simulink model "PropulsionTest"  (R2017b)
settings: Solver=FixedStepAuto  StartTime=0.0  StopTime=100*24*60*60  FixedStep=.2  RelTol=1e-3
model workspace: external: MATLAB File C:\Users\Justin\Documents\00 MEng Project\PAN_ADCS\initialization\simulink_workspace_init.m (data not in the file)
undefined symbols (not defined in the file): Imp_max, Imp_min, init, K_F, L_F, m_follower, match_tol, muE, ontime_max, ontime_min, Thrust_max, Thrust_min
libraries: hEemethod x8, vrlib x2, dspsigattribs x1
(part 2 of 2)

== matlab function PropulsionTest/Position and Velocity to Desired Attitude in Quat/dcm2quat ==
  data: DCM_be input; q output; tr output; q_prev input; flag output
function [q, tr, flag] = fcn(DCM_be,q_prev)
tr= DCM_be(1,1) + DCM_be(2,2) + DCM_be(3,3);
flag=[0 1];
if (tr > 0)
    S= sqrt(1+tr)*2;
    q4= 0.25 * S;
    q1= (DCM_be(3,2)-DCM_be(2,3))/S;
    q2= (DCM_be(1,3)-DCM_be(3,1))/S;
    q3= (DCM_be(2,1)-DCM_be(1,2))/S;
    q=[q1;q2;q3;q4];
    flag(1)=1;
    
elseif ((DCM_be(1,1)>DCM_be(2,2)) && (DCM_be(1,1)>DCM_be(3,3)))
    S= sqrt(1+DCM_be(1,1)-DCM_be(2,2)-DCM_be(3,3))*2;
    q4= (DCM_be(3,2)-DCM_be(2,3))/S;
    q1= 0.25*S;
    q2= (DCM_be(1,2)+DCM_be(2,1))/S;
    q3= (DCM_be(1,3)+DCM_be(3,1))/S;
    flag(1)=2;
    q=[q1;q2;q3;q4];
elseif (DCM_be(2,2)>DCM_be(3,3))
    S= sqrt(1+DCM_be(2,2)-DCM_be(1,1)-DCM_be(3,3))*2;
    q4= (DCM_be(1,3)-DCM_be(3,1))/S;
    q1= (DCM_be(1,2)+DCM_be(2,1))/S;
    q2= 0.25*S;
    q3= (DCM_be(2,3)+DCM_be(3,2))/S;
    flag(1)=3;
    q=[q1;q2;q3;q4];
else
    S= sqrt(1+DCM_be(3,3)-DCM_be(1,1)-DCM_be(2,2))*2;
    q4= (DCM_be(2,1)-DCM_be(1,2))/S;
    q1= (DCM_be(1,3)+DCM_be(3,1))/S;
    q2= (DCM_be(2,3)+DCM_be(3,2))/S;
    q3= 0.25*S;
    flag(1)=4;
    q=[q1;q2;q3;q4];
end


if  (flag(2)*sign(q(1))*sign(q_prev(1))==-1 && q(1)*q(1)>1e-8) || ...
    (flag(2)*sign(q(2))*sign(q_prev(2))==-1 && q(2)*q(2)>1e-8) || ...
    (flag(2)*sign(q(3))*sign(q_prev(3))==-1 && q(3)*q(3)>1e-8)
    %sign(q_prev(1))==0 || ...
    %sign(q_prev(2))==0 || ...
    %sign(q_prev(3))==0
    
    flag(2)=flag(2)*-1;
end
if flag(2)==-1
    q=-q;
end

== matlab function PropulsionTest/Subsystem/Propulsion/MATLAB Function ==
  data: Thrust_vectors output; Target input; onVec output
%%%Thrust Vector Calculations

%  Input: Vectorized Impulse Requirement (Target) [N*s], The Thrust Per Nozzle [N], and the thrust vectors on
%  the current nozzle block (Thrust_vectors, thought this is taken from
%  another function)

%  Output: Thruster On-time vector for the 3 main thrusters, the numbers of
%  the three main thrusters, the on time in terms of thrusters 1,2,3,4

% UNITS of this code is impulse, we take the force vectors of the nozzles
% then scale them accordingly
function [Thrust_vectors, onVec] = get_thruster_onTimes(Target)
%function [t_vector1stage, Best_3_names, onVec] = get_thruster_onTimes(Target,Thrust_per_nozzle)
    % check the input arguments
    [r,c] = size(Target);
    if r~=3 || c~=1
        error('Function argument must be a 3x1 vector')
    end
    % generate the thrust vectors based on the specific nozzle block and
    % the thrust measured per nozzle 
    
    %%% IMPUT THRUST PER NOZZLE %%%
    Thrust_vectors= zeros(3,4);
    Thrust_per_nozzle = 16E-3; %N
    [Thrust_vectors,~] = Generate_Thrust_Vectors(Thrust_per_nozzle); % generates 4x3 matrix 
    
        % determines thrust vectors to be used as a basis in the
        % firing
        angles = zeros(1,4);
        
        % check the angles to each thruster vector
        for i = 1:4 
            angles(i) = acos(dot(Thrust_vectors(:,i),Target)/(norm(Thrust_vectors(:,i))*norm(Target)));
            
        end

        [~,Indices] = sort(angles);
        Best_3_vectors = Thrust_vectors(:,Indices(1:3)); % loads the thruster's vectors
%         Best_2_vectors = Thrust_vectors(:,Indices(1:2));
%         Best_vector = Thrust_vectors(:,Indices(1));
        
        Best_3_names = [0 0 0];
        Best_3_names(1:3) = Indices(1:3); % loads names of the thrusters

        
   % generate on times (2 different methods)
   
   % method 1: 1 stage - 3 thrusters fire in one go, but for different
   % times each, the time vector t_vector1stage gives the thrust for the
   % associated thruster
        
        % x = A\b solves the system of linear equations A*x = b
        t_vector1stage = Best_3_vectors \ Target;

        % remove on_vectors with magnitude <2ms
        for i =1:length(t_vector1stage)
            if t_vector1stage(i) <2E-3 % 2 milliseconds is the min for fire
                t_vector1stage(i) = 0; % reset to zero
            end  
        end
        
        % get the on vector in terms of the nozzles in order
        onVec = zeros(1,4);
        for i = 1:3 % 3 is the number of nozzles given fire orders
            for j = 1:4 % 4 is the number of possible nozzles
                if Best_3_names(i)==j
                   onVec(j) = t_vector1stage(i);
                end
            end

        end
    
        
        
%%%%% METHOD 2 not used as it costs more in terms of opening and closing nozzles and uses the exact same amount of fuel         
%    % method 2: 3 stage
% 
%         bigMat = [ sum(Best_3_vectors,2), sum(Best_2_vectors,2), Best_vector ]; % establishes a vector for three stages with first column as (v1+v2+v3) seoncd (v1+v2), third v1
%         t_vector3stage = bigMat \ Target;


end

%%%Calculate Nozzle Vectors 

function [Thrust_vectors,vectors_unit] = Generate_Thrust_Vectors(Thrust_per_nozzle)

% defined the nozzle block in CAD as Nozzle1, note that each has the
% following sign convention relative to full sat coordinate sytem:
    % Nozzle1:-x+y-z, Nozzle2:+x,-y,-z, Nozzle3:-x,-y,+z, Nozzle4:+x+y+z

% measure the end of the nozzle point in CAD referenced to the Coordinate
% System 2 placed at the hypothetical center of mass of the propulsion
% system in nozzle CAD file, place magnitude of each axis below:

%%% INPUT MEASUREMANTS FROM CADS %%%
magx = 33.93;
magy = 48.73;
magz = 37.172861;
mag_vector = [magx; magy; magz];

% make the vector magnitudes into magnitudes for unit vector
vectors_unit = [magx/norm(mag_vector); magy/norm(mag_vector); magz/norm(mag_vector)];
% scale unit vector by the magnitude of the thrust vector
mag_vector_scaled_thrust = vectors_unit*Thrust_per_nozzle;
% make the unit vectors for each thruster using sign changes
Nozzle1 = [-mag_vector_scaled_thrust(1);+mag_vector_scaled_thrust(2);-mag_vector_scaled_thrust(3)];
Nozzle2 = [+mag_vector_scaled_thrust(1);-mag_vector_scaled_thrust(2);-mag_vector_scaled_thrust(3)];
Nozzle3 = [-mag_vector_scaled_thrust(1);-mag_vector_scaled_thrust(2);+mag_vector_scaled_thrust(3)];
Nozzle4 = [+mag_vector_scaled_thrust(1);+mag_vector_scaled_thrust(2);+mag_vector_scaled_thrust(3)];

Thrust_vectors = [Nozzle1 Nozzle2 Nozzle3 Nozzle4]; % has the thust vector for each nozzle taking into account thrust per nozzle

end
